simulink library "CurrentLoop_Lib"  (R2023a)
settings: Solver=VariableStepAuto  StartTime=0.0  StopTime=10.0  RelTol=1e-3
undefined symbols (not defined in the file): Ki_d, Ki_q, Kp_d, Kp_q, Ld, Lq
settings Model: Creator=HP  LastModifiedBy=HP

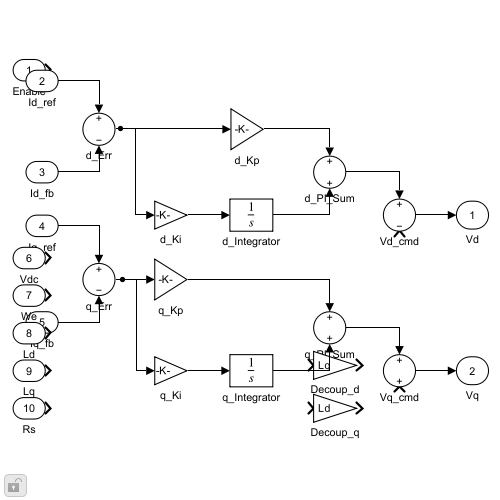
[thumbnail: Simulink's stored preview of the top-level diagram]
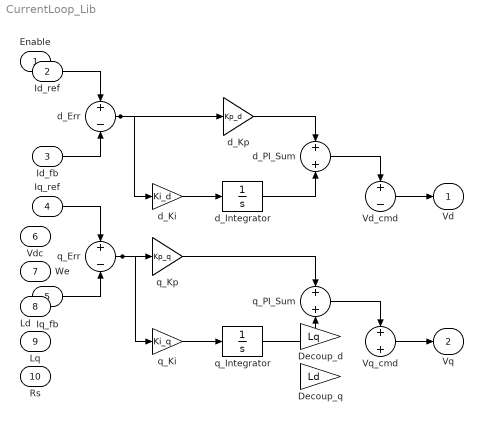
== system CurrentLoop_Lib ==
  Enable : Inport
  Id_ref : Inport  Port=2
  Id_fb : Inport  Port=3
  Iq_ref : Inport  Port=4
  Iq_fb : Inport  Port=5
  Vdc : Inport  Port=6
  We : Inport  Port=7
  Ld : Inport  Port=8
  Lq : Inport  Port=9
  Rs : Inport  Port=10
  Decoup_d : Gain  Gain=Lq
  Decoup_q : Gain  Gain=Ld
  Vd_cmd : Sum  Inputs=+-
  Vq_cmd : Sum
  d_Err : Sum  Inputs=+-
  d_Integrator : Integrator
  d_Ki : Gain  Gain=Ki_d
  d_Kp : Gain  Gain=Kp_d
  d_PI_Sum : Sum
  q_Err : Sum  Inputs=+-
  q_Integrator : Integrator
  q_Ki : Gain  Gain=Ki_q
  q_Kp : Gain  Gain=Kp_q
  q_PI_Sum : Sum
  Vd : Outport
  Vq : Outport  Port=2
  wires:
  Iq_ref/1 -> q_Err/1
  q_Ki/1 -> q_Integrator/1
  Id_fb/1 -> d_Err/2
  Id_ref/1 -> d_Err/1
  d_Integrator/1 -> d_PI_Sum/2
  Iq_fb/1 -> q_Err/2
  q_Err/1 -> q_Kp/1, q_Ki/1
  q_Kp/1 -> q_PI_Sum/1
  d_Err/1 -> d_Kp/1, d_Ki/1
  d_Ki/1 -> d_Integrator/1
  d_Kp/1 -> d_PI_Sum/1
  q_Integrator/1 -> q_PI_Sum/2
  d_PI_Sum/1 -> Vd_cmd/1
  q_PI_Sum/1 -> Vq_cmd/1
  Vd_cmd/1 -> Vd/1
  Vq_cmd/1 -> Vq/1
